simulink library "InfrastructureVariants_CL"  (R2020a)
settings: Solver=VariableStepAuto  StartTime=0.0  StopTime=10.0  RelTol=1e-3
undefined symbols (not defined in the file): Buffer, ENV, Int, Int_ran, route, TRAN, VEH
(part 1 of 2)
settings Model: Creator=John Jr  LastModifiedBy=John Jr
settings DataIOCC: ReturnWorkspaceOutputs=off
settings DebuggingCC: ArithmeticOperatorsInVariantConditions=warning
settings SFSimCC: CustomCodeUndefinedFunction=UseInterfaceOnly

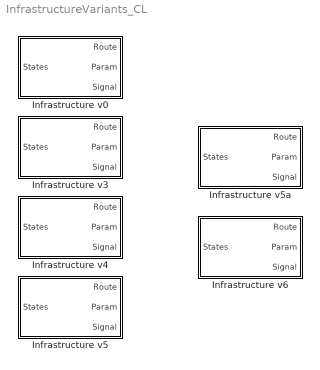
== system InfrastructureVariants_CL ==
  Infrastructure v0 : Subsystem
      mask Display:
      | patch([0 1 1 0], [0 0 1 1],[1 .8 1])
      | 
      | port_label('input',1,'States')
      | 
      | port_label('output',1,'Route')
      | port_label('output',2,'Param')
      | port_label('output',3,'Signal')
  Infrastructure v3 : Subsystem
      mask Display:
      | patch([0 1 1 0], [0 0 1 1],[1 .8 1])
      | 
      | port_label('input',1,'States')
      | 
      | port_label('output',1,'Route')
      | port_label('output',2,'Param')
      | port_label('output',3,'Signal')
  Infrastructure v4 : Subsystem
      mask Display:
      | patch([0 1 1 0], [0 0 1 1],[1 .8 1])
      | 
      | port_label('input',1,'States')
      | 
      | port_label('output',1,'Route')
      | port_label('output',2,'Param')
      | port_label('output',3,'Signal')
  Infrastructure v5 : Subsystem
      mask Display:
      | patch([0 1 1 0], [0 0 1 1],[1 .8 1])
      | 
      | port_label('input',1,'States')
      | 
      | port_label('output',1,'Route')
      | port_label('output',2,'Param')
      | port_label('output',3,'Signal')
  Infrastructure v5a : Subsystem
      mask Display:
      | patch([0 1 1 0], [0 0 1 1],[1 .8 1])
      | 
      | port_label('input',1,'States')
      | 
      | port_label('output',1,'Route')
      | port_label('output',2,'Param')
      | port_label('output',3,'Signal')
  Infrastructure v6 : Subsystem
      mask Display:
      | patch([0 1 1 0], [0 0 1 1],[1 .8 1])
      | 
      | port_label('input',1,'States')
      | 
      | port_label('output',1,'Route')
      | port_label('output',2,'Param')
      | port_label('output',3,'Signal')

== system InfrastructureVariants_CL/Infrastructure v0 ==
  States : Inport
  Route Generator : Subsystem
  Signal Info v5 : Subsystem
      mask Display:
      | patch([0 1 1 0], [0 0 1 1],[.8 1 1])
      | 
      | port_label('input',1,'States')
      | 
      | port_label('output',1,'Signal')
  Veh Param : Subsystem
  Route : Outport  VectorParamsAs1DForOutWhenUnconnected=off
  Param : Outport  Port=2  VectorParamsAs1DForOutWhenUnconnected=off
  Signal : Outport  Port=3  VectorParamsAs1DForOutWhenUnconnected=off
  wires:
  States/1 -> Signal Info v5/1(In1)
  Route Generator/1(Route Info) -> Route/1
  Veh Param/1(Param) -> Param/1
  Signal Info v5/1(Out1) -> Signal/1

== system InfrastructureVariants_CL/Infrastructure v3 ==
  States : Inport
  Route Generator : Subsystem
  Signal Info v3 : Subsystem
      mask Display:
      | patch([0 1 1 0], [0 0 1 1],[.8 1 1])
      | 
      | port_label('input',1,'States')
      | 
      | port_label('output',1,'Signal')
  Veh Param : Subsystem
  Route : Outport  VectorParamsAs1DForOutWhenUnconnected=off
  Param : Outport  Port=2  VectorParamsAs1DForOutWhenUnconnected=off
  Signal : Outport  Port=3  VectorParamsAs1DForOutWhenUnconnected=off
  wires:
  States/1 -> Signal Info v3/1(In1)
  Route Generator/1(Route Info) -> Route/1
  Veh Param/1(Param) -> Param/1
  Signal Info v3/1(Out1) -> Signal/1

== system InfrastructureVariants_CL/Infrastructure v4 ==
  States : Inport
  Route Generator : Subsystem
  Signal Info v4 : Subsystem
      mask Display:
      | patch([0 1 1 0], [0 0 1 1],[.8 1 1])
      | 
      | port_label('input',1,'States')
      | 
      | port_label('output',1,'Signal')
  Veh Param : Subsystem
  Route : Outport  VectorParamsAs1DForOutWhenUnconnected=off
  Param : Outport  Port=2  VectorParamsAs1DForOutWhenUnconnected=off
  Signal : Outport  Port=3  VectorParamsAs1DForOutWhenUnconnected=off
  wires:
  States/1 -> Signal Info v4/1(In1)
  Route Generator/1(Route Info) -> Route/1
  Veh Param/1(Param) -> Param/1
  Signal Info v4/1(Out1) -> Signal/1

== system InfrastructureVariants_CL/Infrastructure v5 ==
  States : Inport
  Route Generator : Subsystem
  Signal Info v5 : Subsystem
      mask Display:
      | patch([0 1 1 0], [0 0 1 1],[.8 1 1])
      | 
      | port_label('input',1,'States')
      | 
      | port_label('output',1,'Signal')
  Veh Param : Subsystem
  Route : Outport  VectorParamsAs1DForOutWhenUnconnected=off
  Param : Outport  Port=2  VectorParamsAs1DForOutWhenUnconnected=off
  Signal : Outport  Port=3  VectorParamsAs1DForOutWhenUnconnected=off
  wires:
  States/1 -> Signal Info v5/1(In1)
  Route Generator/1(Route Info) -> Route/1
  Veh Param/1(Param) -> Param/1
  Signal Info v5/1(Out1) -> Signal/1

== system InfrastructureVariants_CL/Infrastructure v5a ==
  States : Inport
  Route Generator : Subsystem
  Signal Info v5a : Subsystem
      mask Display:
      | patch([0 1 1 0], [0 0 1 1],[.8 1 1])
      | 
      | port_label('input',1,'States')
      | 
      | port_label('output',1,'Signal')
  Veh Param : Subsystem
  Route : Outport  VectorParamsAs1DForOutWhenUnconnected=off
  Param : Outport  Port=2  VectorParamsAs1DForOutWhenUnconnected=off
  Signal : Outport  Port=3  VectorParamsAs1DForOutWhenUnconnected=off
  wires:
  States/1 -> Signal Info v5a/1(In1)
  Route Generator/1(Route Info) -> Route/1
  Veh Param/1(Param) -> Param/1
  Signal Info v5a/1(Out1) -> Signal/1

== system InfrastructureVariants_CL/Infrastructure v6 ==
  States : Inport
  Route Generator : Subsystem
  Signal Info v5 : Subsystem
      mask Display:
      | patch([0 1 1 0], [0 0 1 1],[.8 1 1])
      | 
      | port_label('input',1,'States')
      | 
      | port_label('output',1,'Signal')
  Veh Param : Subsystem
  Route : Outport  VectorParamsAs1DForOutWhenUnconnected=off
  Param : Outport  Port=2  VectorParamsAs1DForOutWhenUnconnected=off
  Signal : Outport  Port=3  VectorParamsAs1DForOutWhenUnconnected=off
  wires:
  States/1 -> Signal Info v5/1(In1)
  Route Generator/1(Route Info) -> Route/1
  Veh Param/1(Param) -> Param/1
  Signal Info v5/1(Out1) -> Signal/1

== system InfrastructureVariants_CL/Infrastructure v0/Route Generator ==
  Constant1 : Constant  Value=route
  Route Info : Outport  VectorParamsAs1DForOutWhenUnconnected=off
  wires:
  Constant1/1 -> Route Info/1  "route"

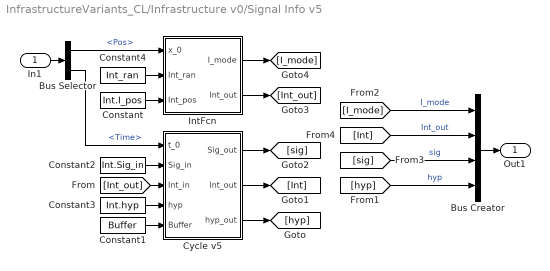
== system InfrastructureVariants_CL/Infrastructure v0/Signal Info v5 ==
  In1 : Inport
  Bus Creator : BusCreator  Inputs=4
  Bus Selector : BusSelector  OutputSignals=Pos,Time
  Constant : Constant  Value=Int.I_pos
  Constant1 : Constant  Value=Buffer
  Constant2 : Constant  Value=Int.Sig_in
  Constant3 : Constant  Value=Int.hyp
  Constant4 : Constant  Value=Int_ran
  Cycle v5 : MATLAB Function  TreatAsAtomicUnit=on
  IntFcn : MATLAB Function  TreatAsAtomicUnit=on
  Out1 : Outport  VectorParamsAs1DForOutWhenUnconnected=off
  wires:
  Constant1/1 -> Cycle v5/5(Buffer)
  Cycle v5/3(hyp_out) -> [hyp]
  Cycle v5/2(Int_out) -> [Int]
  Cycle v5/1(Sig_out) -> [sig]
  [sig] -> Bus Creator/3  "sig"
  [hyp] -> Bus Creator/4  "hyp"
  Bus Creator/1 -> Out1/1
  Constant3/1 -> Cycle v5/4(hyp)
  Constant4/1 -> IntFcn/2(Int_ran)
  [Int_out] -> Cycle v5/3(Int_in)
  IntFcn/2(Int_out) -> [Int_out]
  [Int] -> Bus Creator/2  "Int_out"
  Constant/1 -> IntFcn/3(Int_pos)
  IntFcn/1(I_mode) -> [I_mode]
  [I_mode] -> Bus Creator/1  "I_mode"
  Constant2/1 -> Cycle v5/2(Sig_in)
  In1/1 -> Bus Selector/1
  Bus Selector/1 -> IntFcn/1(x_0)  "<Pos>"
  Bus Selector/2 -> Cycle v5/1(t_0)  "<Time>"

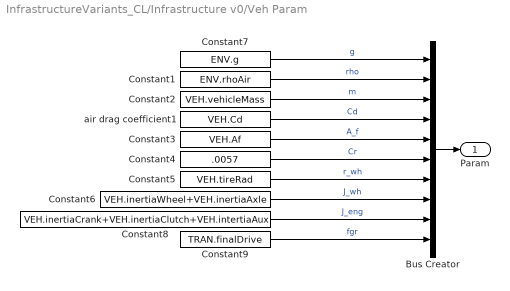
== system InfrastructureVariants_CL/Infrastructure v0/Veh Param ==
  Bus Creator : BusCreator  Inputs=10
  Constant1 : Constant  Value=ENV.rhoAir
  Constant2 : Constant  Value=VEH.vehicleMass
  Constant3 : Constant  Value=VEH.Af
  Constant4 : Constant  Value=.0057
  Constant5 : Constant  Value=VEH.tireRad
  Constant6 : Constant  Value=VEH.inertiaWheel+VEH.inertiaAxle
  Constant7 : Constant  Value=ENV.g
  Constant8 : Constant  Value=VEH.inertiaCrank+VEH.inertiaClutch+VEH.intertiaAux
  Constant9 : Constant  Value=TRAN.finalDrive
  air drag coefficient1 : Constant  Value=VEH.Cd
  Param : Outport  VectorParamsAs1DForOutWhenUnconnected=off
  wires:
  Bus Creator/1 -> Param/1
  Constant7/1 -> Bus Creator/1  "g"
  Constant1/1 -> Bus Creator/2  "rho"
  Constant2/1 -> Bus Creator/3  "m"
  Constant3/1 -> Bus Creator/5  "A_f"
  Constant4/1 -> Bus Creator/6  "Cr"
  Constant5/1 -> Bus Creator/7  "r_wh"
  Constant9/1 -> Bus Creator/10  "fgr"
  air drag coefficient1/1 -> Bus Creator/4  "Cd"
  Constant6/1 -> Bus Creator/8  "J_wh"
  Constant8/1 -> Bus Creator/9  "J_eng"

== system InfrastructureVariants_CL/Infrastructure v3/Route Generator ==
  Constant1 : Constant  Value=route
  Route Info : Outport  VectorParamsAs1DForOutWhenUnconnected=off
  wires:
  Constant1/1 -> Route Info/1  "route"

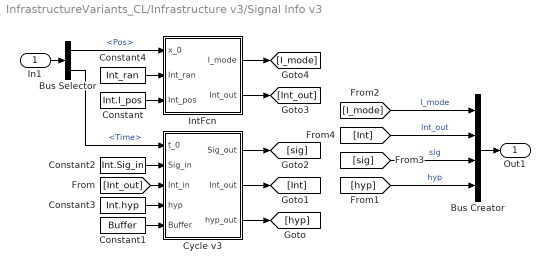
== system InfrastructureVariants_CL/Infrastructure v3/Signal Info v3 ==
  In1 : Inport
  Bus Creator : BusCreator  Inputs=4
  Bus Selector : BusSelector  OutputSignals=Pos,Time
  Constant : Constant  Value=Int.I_pos
  Constant1 : Constant  Value=Buffer
  Constant2 : Constant  Value=Int.Sig_in
  Constant3 : Constant  Value=Int.hyp
  Constant4 : Constant  Value=Int_ran
  Cycle v3 : MATLAB Function  TreatAsAtomicUnit=on
  IntFcn : MATLAB Function  TreatAsAtomicUnit=on
  Out1 : Outport  VectorParamsAs1DForOutWhenUnconnected=off
  wires:
  Constant1/1 -> Cycle v3/5(Buffer)
  Cycle v3/3(hyp_out) -> [hyp]
  Cycle v3/2(Int_out) -> [Int]
  Cycle v3/1(Sig_out) -> [sig]
  [sig] -> Bus Creator/3  "sig"
  [hyp] -> Bus Creator/4  "hyp"
  Bus Creator/1 -> Out1/1
  Constant3/1 -> Cycle v3/4(hyp)
  Constant4/1 -> IntFcn/2(Int_ran)
  [Int_out] -> Cycle v3/3(Int_in)
  IntFcn/2(Int_out) -> [Int_out]
  [Int] -> Bus Creator/2  "Int_out"
  Constant/1 -> IntFcn/3(Int_pos)
  IntFcn/1(I_mode) -> [I_mode]
  [I_mode] -> Bus Creator/1  "I_mode"
  Constant2/1 -> Cycle v3/2(Sig_in)
  In1/1 -> Bus Selector/1
  Bus Selector/1 -> IntFcn/1(x_0)  "<Pos>"
  Bus Selector/2 -> Cycle v3/1(t_0)  "<Time>"

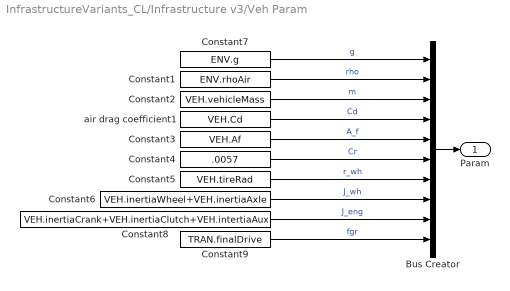
== system InfrastructureVariants_CL/Infrastructure v3/Veh Param ==
  Bus Creator : BusCreator  Inputs=10
  Constant1 : Constant  Value=ENV.rhoAir
  Constant2 : Constant  Value=VEH.vehicleMass
  Constant3 : Constant  Value=VEH.Af
  Constant4 : Constant  Value=.0057
  Constant5 : Constant  Value=VEH.tireRad
  Constant6 : Constant  Value=VEH.inertiaWheel+VEH.inertiaAxle
  Constant7 : Constant  Value=ENV.g
  Constant8 : Constant  Value=VEH.inertiaCrank+VEH.inertiaClutch+VEH.intertiaAux
  Constant9 : Constant  Value=TRAN.finalDrive
  air drag coefficient1 : Constant  Value=VEH.Cd
  Param : Outport  VectorParamsAs1DForOutWhenUnconnected=off
  wires:
  Bus Creator/1 -> Param/1
  Constant7/1 -> Bus Creator/1  "g"
  Constant1/1 -> Bus Creator/2  "rho"
  Constant2/1 -> Bus Creator/3  "m"
  Constant3/1 -> Bus Creator/5  "A_f"
  Constant4/1 -> Bus Creator/6  "Cr"
  Constant5/1 -> Bus Creator/7  "r_wh"
  Constant9/1 -> Bus Creator/10  "fgr"
  air drag coefficient1/1 -> Bus Creator/4  "Cd"
  Constant6/1 -> Bus Creator/8  "J_wh"
  Constant8/1 -> Bus Creator/9  "J_eng"

== system InfrastructureVariants_CL/Infrastructure v4/Route Generator ==
  Constant1 : Constant  Value=route
  Route Info : Outport  VectorParamsAs1DForOutWhenUnconnected=off
  wires:
  Constant1/1 -> Route Info/1  "route"

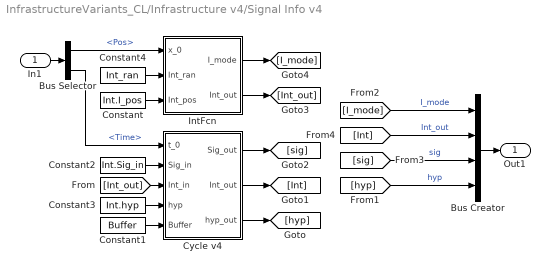
== system InfrastructureVariants_CL/Infrastructure v4/Signal Info v4 ==
  In1 : Inport
  Bus Creator : BusCreator  Inputs=4
  Bus Selector : BusSelector  OutputSignals=Pos,Time
  Constant : Constant  Value=Int.I_pos
  Constant1 : Constant  Value=Buffer
  Constant2 : Constant  Value=Int.Sig_in
  Constant3 : Constant  Value=Int.hyp
  Constant4 : Constant  Value=Int_ran
  Cycle v4 : MATLAB Function  TreatAsAtomicUnit=on
  IntFcn : MATLAB Function  TreatAsAtomicUnit=on
  Out1 : Outport  VectorParamsAs1DForOutWhenUnconnected=off
  wires:
  Constant1/1 -> Cycle v4/5(Buffer)
  Cycle v4/3(hyp_out) -> [hyp]
  Cycle v4/2(Int_out) -> [Int]
  Cycle v4/1(Sig_out) -> [sig]
  [sig] -> Bus Creator/3  "sig"
  [hyp] -> Bus Creator/4  "hyp"
  Bus Creator/1 -> Out1/1
  Constant3/1 -> Cycle v4/4(hyp)
  Constant4/1 -> IntFcn/2(Int_ran)
  [Int_out] -> Cycle v4/3(Int_in)
  IntFcn/2(Int_out) -> [Int_out]
  [Int] -> Bus Creator/2  "Int_out"
  Constant/1 -> IntFcn/3(Int_pos)
  IntFcn/1(I_mode) -> [I_mode]
  [I_mode] -> Bus Creator/1  "I_mode"
  Constant2/1 -> Cycle v4/2(Sig_in)
  In1/1 -> Bus Selector/1
  Bus Selector/1 -> IntFcn/1(x_0)  "<Pos>"
  Bus Selector/2 -> Cycle v4/1(t_0)  "<Time>"

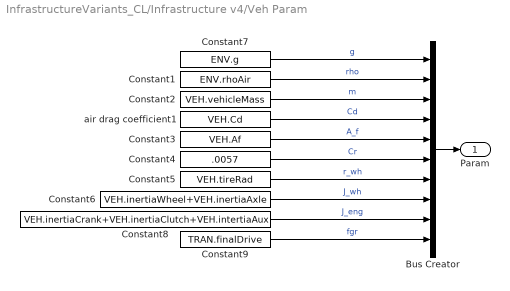
== system InfrastructureVariants_CL/Infrastructure v4/Veh Param ==
  Bus Creator : BusCreator  Inputs=10
  Constant1 : Constant  Value=ENV.rhoAir
  Constant2 : Constant  Value=VEH.vehicleMass
  Constant3 : Constant  Value=VEH.Af
  Constant4 : Constant  Value=.0057
  Constant5 : Constant  Value=VEH.tireRad
  Constant6 : Constant  Value=VEH.inertiaWheel+VEH.inertiaAxle
  Constant7 : Constant  Value=ENV.g
  Constant8 : Constant  Value=VEH.inertiaCrank+VEH.inertiaClutch+VEH.intertiaAux
  Constant9 : Constant  Value=TRAN.finalDrive
  air drag coefficient1 : Constant  Value=VEH.Cd
  Param : Outport  VectorParamsAs1DForOutWhenUnconnected=off
  wires:
  Bus Creator/1 -> Param/1
  Constant7/1 -> Bus Creator/1  "g"
  Constant1/1 -> Bus Creator/2  "rho"
  Constant2/1 -> Bus Creator/3  "m"
  Constant3/1 -> Bus Creator/5  "A_f"
  Constant4/1 -> Bus Creator/6  "Cr"
  Constant5/1 -> Bus Creator/7  "r_wh"
  Constant9/1 -> Bus Creator/10  "fgr"
  air drag coefficient1/1 -> Bus Creator/4  "Cd"
  Constant6/1 -> Bus Creator/8  "J_wh"
  Constant8/1 -> Bus Creator/9  "J_eng"

== system InfrastructureVariants_CL/Infrastructure v5/Route Generator ==
  Constant1 : Constant  Value=route
  Route Info : Outport  VectorParamsAs1DForOutWhenUnconnected=off
  wires:
  Constant1/1 -> Route Info/1  "route"

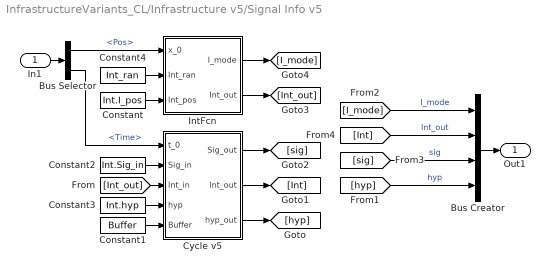
== system InfrastructureVariants_CL/Infrastructure v5/Signal Info v5 ==
  In1 : Inport
  Bus Creator : BusCreator  Inputs=4
  Bus Selector : BusSelector  OutputSignals=Pos,Time
  Constant : Constant  Value=Int.I_pos
  Constant1 : Constant  Value=Buffer
  Constant2 : Constant  Value=Int.Sig_in
  Constant3 : Constant  Value=Int.hyp
  Constant4 : Constant  Value=Int_ran
  Cycle v5 : MATLAB Function  TreatAsAtomicUnit=on
  IntFcn : MATLAB Function  TreatAsAtomicUnit=on
  Out1 : Outport  VectorParamsAs1DForOutWhenUnconnected=off
  wires:
  Constant1/1 -> Cycle v5/5(Buffer)
  Cycle v5/3(hyp_out) -> [hyp]
  Cycle v5/2(Int_out) -> [Int]
  Cycle v5/1(Sig_out) -> [sig]
  [sig] -> Bus Creator/3  "sig"
  [hyp] -> Bus Creator/4  "hyp"
  Bus Creator/1 -> Out1/1
  Constant3/1 -> Cycle v5/4(hyp)
  Constant4/1 -> IntFcn/2(Int_ran)
  [Int_out] -> Cycle v5/3(Int_in)
  IntFcn/2(Int_out) -> [Int_out]
  [Int] -> Bus Creator/2  "Int_out"
  Constant/1 -> IntFcn/3(Int_pos)
  IntFcn/1(I_mode) -> [I_mode]
  [I_mode] -> Bus Creator/1  "I_mode"
  Constant2/1 -> Cycle v5/2(Sig_in)
  In1/1 -> Bus Selector/1
  Bus Selector/1 -> IntFcn/1(x_0)  "<Pos>"
  Bus Selector/2 -> Cycle v5/1(t_0)  "<Time>"

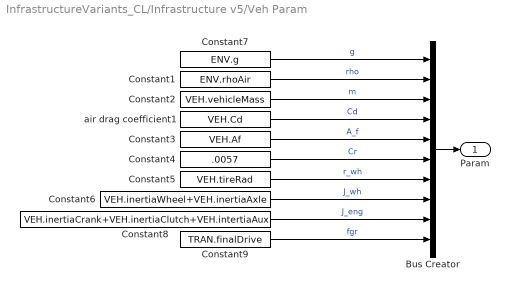
== system InfrastructureVariants_CL/Infrastructure v5/Veh Param ==
  Bus Creator : BusCreator  Inputs=10
  Constant1 : Constant  Value=ENV.rhoAir
  Constant2 : Constant  Value=VEH.vehicleMass
  Constant3 : Constant  Value=VEH.Af
  Constant4 : Constant  Value=.0057
  Constant5 : Constant  Value=VEH.tireRad
  Constant6 : Constant  Value=VEH.inertiaWheel+VEH.inertiaAxle
  Constant7 : Constant  Value=ENV.g
  Constant8 : Constant  Value=VEH.inertiaCrank+VEH.inertiaClutch+VEH.intertiaAux
  Constant9 : Constant  Value=TRAN.finalDrive
  air drag coefficient1 : Constant  Value=VEH.Cd
  Param : Outport  VectorParamsAs1DForOutWhenUnconnected=off
  wires:
  Bus Creator/1 -> Param/1
  Constant7/1 -> Bus Creator/1  "g"
  Constant1/1 -> Bus Creator/2  "rho"
  Constant2/1 -> Bus Creator/3  "m"
  Constant3/1 -> Bus Creator/5  "A_f"
  Constant4/1 -> Bus Creator/6  "Cr"
  Constant5/1 -> Bus Creator/7  "r_wh"
  Constant9/1 -> Bus Creator/10  "fgr"
  air drag coefficient1/1 -> Bus Creator/4  "Cd"
  Constant6/1 -> Bus Creator/8  "J_wh"
  Constant8/1 -> Bus Creator/9  "J_eng"

== system InfrastructureVariants_CL/Infrastructure v5a/Route Generator ==
  Constant1 : Constant  Value=route
  Route Info : Outport  VectorParamsAs1DForOutWhenUnconnected=off
  wires:
  Constant1/1 -> Route Info/1  "route"

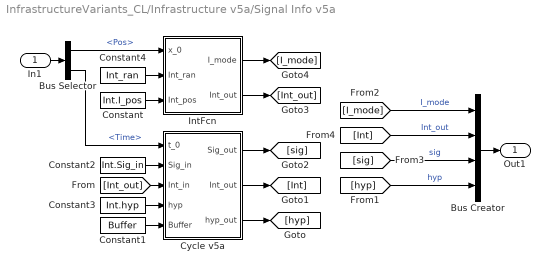
== system InfrastructureVariants_CL/Infrastructure v5a/Signal Info v5a ==
  In1 : Inport
  Bus Creator : BusCreator  Inputs=4
  Bus Selector : BusSelector  OutputSignals=Pos,Time
  Constant : Constant  Value=Int.I_pos
  Constant1 : Constant  Value=Buffer
  Constant2 : Constant  Value=Int.Sig_in
  Constant3 : Constant  Value=Int.hyp
  Constant4 : Constant  Value=Int_ran
  Cycle v5a : MATLAB Function  TreatAsAtomicUnit=on
  IntFcn : MATLAB Function  TreatAsAtomicUnit=on
  Out1 : Outport  VectorParamsAs1DForOutWhenUnconnected=off
  wires:
  Constant1/1 -> Cycle v5a/5(Buffer)
  Cycle v5a/3(hyp_out) -> [hyp]
  Cycle v5a/2(Int_out) -> [Int]
  Cycle v5a/1(Sig_out) -> [sig]
  [sig] -> Bus Creator/3  "sig"
  [hyp] -> Bus Creator/4  "hyp"
  Bus Creator/1 -> Out1/1
  Constant3/1 -> Cycle v5a/4(hyp)
  Constant4/1 -> IntFcn/2(Int_ran)
  [Int_out] -> Cycle v5a/3(Int_in)
  IntFcn/2(Int_out) -> [Int_out]
  [Int] -> Bus Creator/2  "Int_out"
  Constant/1 -> IntFcn/3(Int_pos)
  IntFcn/1(I_mode) -> [I_mode]
  [I_mode] -> Bus Creator/1  "I_mode"
  Constant2/1 -> Cycle v5a/2(Sig_in)
  In1/1 -> Bus Selector/1
  Bus Selector/1 -> IntFcn/1(x_0)  "<Pos>"
  Bus Selector/2 -> Cycle v5a/1(t_0)  "<Time>"

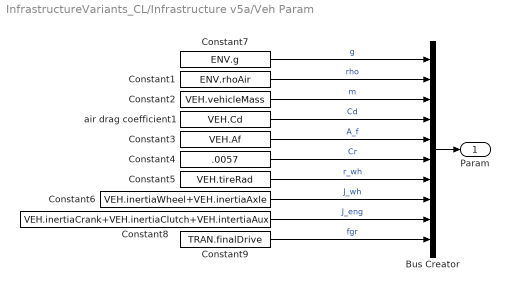
== system InfrastructureVariants_CL/Infrastructure v5a/Veh Param ==
  Bus Creator : BusCreator  Inputs=10
  Constant1 : Constant  Value=ENV.rhoAir
  Constant2 : Constant  Value=VEH.vehicleMass
  Constant3 : Constant  Value=VEH.Af
  Constant4 : Constant  Value=.0057
  Constant5 : Constant  Value=VEH.tireRad
  Constant6 : Constant  Value=VEH.inertiaWheel+VEH.inertiaAxle
  Constant7 : Constant  Value=ENV.g
  Constant8 : Constant  Value=VEH.inertiaCrank+VEH.inertiaClutch+VEH.intertiaAux
  Constant9 : Constant  Value=TRAN.finalDrive
  air drag coefficient1 : Constant  Value=VEH.Cd
  Param : Outport  VectorParamsAs1DForOutWhenUnconnected=off
  wires:
  Bus Creator/1 -> Param/1
  Constant7/1 -> Bus Creator/1  "g"
  Constant1/1 -> Bus Creator/2  "rho"
  Constant2/1 -> Bus Creator/3  "m"
  Constant3/1 -> Bus Creator/5  "A_f"
  Constant4/1 -> Bus Creator/6  "Cr"
  Constant5/1 -> Bus Creator/7  "r_wh"
  Constant9/1 -> Bus Creator/10  "fgr"
  air drag coefficient1/1 -> Bus Creator/4  "Cd"
  Constant6/1 -> Bus Creator/8  "J_wh"
  Constant8/1 -> Bus Creator/9  "J_eng"

== system InfrastructureVariants_CL/Infrastructure v6/Route Generator ==
  Constant1 : Constant  Value=route
  Route Info : Outport  VectorParamsAs1DForOutWhenUnconnected=off
  wires:
  Constant1/1 -> Route Info/1  "route"

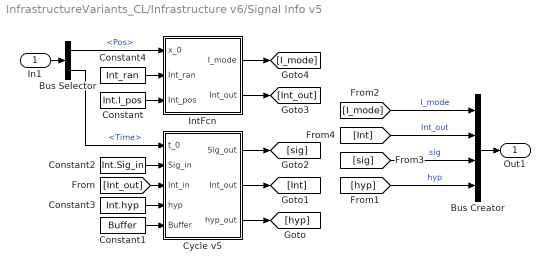
== system InfrastructureVariants_CL/Infrastructure v6/Signal Info v5 ==
  In1 : Inport
  Bus Creator : BusCreator  Inputs=4
  Bus Selector : BusSelector  OutputSignals=Pos,Time
  Constant : Constant  Value=Int.I_pos
  Constant1 : Constant  Value=Buffer
  Constant2 : Constant  Value=Int.Sig_in
  Constant3 : Constant  Value=Int.hyp
  Constant4 : Constant  Value=Int_ran
  Cycle v5 : MATLAB Function  TreatAsAtomicUnit=on
  IntFcn : MATLAB Function  TreatAsAtomicUnit=on
  Out1 : Outport  VectorParamsAs1DForOutWhenUnconnected=off
  wires:
  Constant1/1 -> Cycle v5/5(Buffer)
  Cycle v5/3(hyp_out) -> [hyp]
  Cycle v5/2(Int_out) -> [Int]
  Cycle v5/1(Sig_out) -> [sig]
  [sig] -> Bus Creator/3  "sig"
  [hyp] -> Bus Creator/4  "hyp"
  Bus Creator/1 -> Out1/1
  Constant3/1 -> Cycle v5/4(hyp)
  Constant4/1 -> IntFcn/2(Int_ran)
  [Int_out] -> Cycle v5/3(Int_in)
  IntFcn/2(Int_out) -> [Int_out]
  [Int] -> Bus Creator/2  "Int_out"
  Constant/1 -> IntFcn/3(Int_pos)
  IntFcn/1(I_mode) -> [I_mode]
  [I_mode] -> Bus Creator/1  "I_mode"
  Constant2/1 -> Cycle v5/2(Sig_in)
  In1/1 -> Bus Selector/1
  Bus Selector/1 -> IntFcn/1(x_0)  "<Pos>"
  Bus Selector/2 -> Cycle v5/1(t_0)  "<Time>"

== system InfrastructureVariants_CL/Infrastructure v6/Veh Param ==
  Bus Creator : BusCreator  Inputs=10
  Constant1 : Constant  Value=ENV.rhoAir
  Constant2 : Constant  Value=VEH.vehicleMass
  Constant3 : Constant  Value=VEH.Af
  Constant4 : Constant  Value=.0057
  Constant5 : Constant  Value=VEH.tireRad
  Constant6 : Constant  Value=VEH.inertiaWheel+VEH.inertiaAxle
  Constant7 : Constant  Value=ENV.g
  Constant8 : Constant  Value=VEH.inertiaCrank+VEH.inertiaClutch+VEH.intertiaAux
  Constant9 : Constant  Value=TRAN.finalDrive
  air drag coefficient1 : Constant  Value=VEH.Cd
  Param : Outport  VectorParamsAs1DForOutWhenUnconnected=off
  wires:
  Bus Creator/1 -> Param/1
  Constant7/1 -> Bus Creator/1  "g"
  Constant1/1 -> Bus Creator/2  "rho"
  Constant2/1 -> Bus Creator/3  "m"
  Constant3/1 -> Bus Creator/5  "A_f"
  Constant4/1 -> Bus Creator/6  "Cr"
  Constant5/1 -> Bus Creator/7  "r_wh"
  Constant9/1 -> Bus Creator/10  "fgr"
  air drag coefficient1/1 -> Bus Creator/4  "Cd"
  Constant6/1 -> Bus Creator/8  "J_wh"
  Constant8/1 -> Bus Creator/9  "J_eng"

== matlab function InfrastructureVariants_CL/Infrastructure v6/Signal Info v5/Cycle v5 ==
  data: Sig_out output; Int_out output; t_0 input; Sig_in input; Int_in input; hyp_out output; hyp input; Buffer input
function [Sig_out,Int_out,hyp_out] = fcn(t_0,Sig_in,Int_in,hyp,Buffer)

Int_cur = Int_in(~isnan(Int_in(:,1)),1);        %   Current intersections within communication range
Cs = Sig_in(:,:,1);                             %   s - Signal cycle start times
G = Sig_in(:,:,3);                              %   s - Signal green phase length 
R = Sig_in(:,:,4);                              %   s - Signal red phase length 
Y = Buffer(:,1);                                %   s - Signal yellow length
Rc = Buffer(:,2);                               %   s - Signal red clearance length 
N = 10;                                         %   # of upcoming intersections 
M = 20;                                         %   Size of intersection data queue
idx = zeros(N,1);                               %   Initialize current cycle index vector
Sig_out = NaN*ones(N,M,4);                      %   Initialize cycle length output 
hyp_out = NaN*ones(N,3,2);                      %   Initialize hyperparameter output 
T_0 = NaN*ones(N,1);                            %   Initialize current cycle start time output
L_0 = NaN*ones(N,1);                            %   Initialize light status flag
B_0 = NaN*ones(N,1);                            %   Initialize yellow light length 
for i = 1:length(Int_cur)
    idx(i) = find(Cs(Int_cur(i),:) <= t_0,1,'last');        %   Find current cycle for upcoming intersections 
    tR = Cs(Int_cur(i),idx(i))+G(Int_cur(i),idx(i));        %   s - Time at which light turns red
    tL1 = tR-t_0;                                           %   s - Time left until red
    tL2 = Cs(Int_cur(i),idx(i)+1)-t_0;                      %   s - Time left until green
    if tL1 > Y(Int_cur(i))*2 
        L_0(i) = 0;                                         %   Light is green and time left is unknown 
        Sig_out(i,:,3) = idx(i)-M:idx(i)-1;                 %   Available green phase lengths
        Sig_out(i,:,4) = idx(i)-M:idx(i)-1;                 %   Available red phase lengths
    elseif tL1 <= Y(Int_cur(i))*2 && tL1 > 0
        L_0(i) = 1;                                         %   Light is green and time left is known 
        Sig_out(i,:,3) = idx(i)-M+1:idx(i);                 %   Available green phase lengths
        Sig_out(i,:,4) = idx(i)-M:idx(i)-1;                 %   Available red phase lengths
    elseif tL2 > (Y(Int_cur(i))+Rc(Int_cur(i)))*2 
        L_0(i) = 2;                                         %   Light is red and time left is unknown 
        Sig_out(i,:,3) = idx(i)-M+1:idx(i);                 %   Available green phase lengths
        Sig_out(i,:,4) = idx(i)-M:idx(i)-1;                 %   Available red phase lengths
    else           
        L_0(i) = 3;                                         %   Light is red and time left is known 
        Sig_out(i,:,3) = idx(i)-M+1:idx(i);                 %   Available green phase lengths
        Sig_out(i,:,4) = idx(i)-M+1:idx(i);                 %   Available red phase lengths
    end
    B_0(i) = 2*Y(Int_cur(i));                               %   Yellow light length for upcoming intersections 
    Sig_out(i,:,1) = G(Int_cur(i),Sig_out(i,:,3));          %   Create a vector with the past green phase lengths
    Sig_out(i,:,2) = R(Int_cur(i),Sig_out(i,:,4));          %   Create a vector with the past red phase lengths
    T_0(i) = Cs(Int_cur(i),idx(i));                         %   Current cycle start time
    hypG1 = var(Sig_out(i,:,1));
    hypR1 = var(Sig_out(i,:,2));
    hyp_out(i,:,1) = [hypG1 1 .0625];                       %   Get relevant hyperparameters 
    hyp_out(i,:,2) = [hypR1 1 .0625];                       %   Get relevant hyperparameters 
end
Int_out = [Int_in, T_0, L_0, B_0];                          %   Update intersection variables

== matlab function InfrastructureVariants_CL/Infrastructure v6/Signal Info v5/IntFcn ==
  data: x_0 input; I_mode output; Int_ran input; Int_pos input; Int_out output
function [I_mode,Int_out]  = fcn(x_0,Int_ran,Int_pos)

Int_pos = Int_pos(:,1);                         %   Intersection Positions
[Int_0,~] = find(x_0-Int_pos < 0,1,'first');    %   First intersection within range
[Int_f,~] = find(x_0+Int_ran-Int_pos...         %   Last intersection within range
    > 0,1,'last');
Int_cur = NaN*ones(10,1);                       %   Initialize upcoming intersection vector 
Int_dx = NaN*ones(10,1);                        %   m - Initialize distance to upcoming intersections vector 
Int_gap = NaN*ones(10,1);                       %   m - Initialize distance between intersections vector 
if isempty(Int_0)
    I_mode = 0;                                 %   No upcoming intersection
elseif Int_pos(Int_0(1))-x_0 > Int_ran
    I_mode = 0;                                 %   No upcoming intersection
else
    I_0 = Int_0(1);     I_f = Int_f(1);
    Int_cur(1:I_f-I_0+1,1) = (I_0:I_f)';            %   Upcoming intersections
    I_mode = 1;                                 %   Approaching intersection
    Int_dx(1:I_f-I_0+1,1) = ...                 %   m - Distance to upcoming intersection 
        Int_pos(Int_cur(1:I_f-I_0+1,1))-x_0;
end
Int_gap(1) = Int_dx(1);                         %   m - Distance to first upcoming intersection 
for i = 2:length(Int_gap)
    Int_gap(i) = Int_dx(i)-Int_dx(i-1);         %   m - Distance between further intersections 
end
Int_out = [Int_cur,Int_dx,Int_gap];

== matlab function InfrastructureVariants_CL/Infrastructure v5a/Signal Info v5a/Cycle v5a ==
  data: Sig_out output; Int_out output; t_0 input; Sig_in input; Int_in input; hyp_out output; hyp input; Buffer input
function [Sig_out,Int_out,hyp_out] = fcn(t_0,Sig_in,Int_in,hyp,Buffer)

Int_cur = Int_in(~isnan(Int_in(:,1)),1);        %   Current intersections within communication range
Cs = Sig_in(:,:,1);                             %   s - Signal cycle start times
G = Sig_in(:,:,3);                              %   s - Signal green phase length 
R = Sig_in(:,:,4);                              %   s - Signal red phase length 
Y = Buffer(:,1);                                %   s - Signal yellow length
Rc = Buffer(:,2);                               %   s - Signal red clearance length 
N = 10;                                         %   # of upcoming intersections 
M = 7;                                         %   Size of intersection data queue
idx = zeros(N,1);                               %   Initialize current cycle index vector
Sig_out = NaN*ones(N,M,4);                      %   Initialize cycle length output 
hyp_out = NaN*ones(N,3,2);                      %   Initialize hyperparameter output 
T_0 = NaN*ones(N,1);                            %   Initialize current cycle start time output
L_0 = NaN*ones(N,1);                            %   Initialize light status flag
B_0 = NaN*ones(N,1);                            %   Initialize yellow light length 
for i = 1:length(Int_cur)
    idx(i) = find(Cs(Int_cur(i),:) <= t_0,1,'last');        %   Find current cycle for upcoming intersections 
    B_0(i) = 2*Y(Int_cur(i));                               %   Yellow light length for upcoming intersections 
    Sig_out(i,:,3) = idx(i):idx(i)+M-1;                     %   Available green phase lengths
    Sig_out(i,:,4) = idx(i):idx(i)+M-1;                     %   Available red phase lengths
    Sig_out(i,:,1) = G(Int_cur(i),Sig_out(i,:,3));          %   Create a vector with the past green phase lengths
    Sig_out(i,:,2) = R(Int_cur(i),Sig_out(i,:,4));          %   Create a vector with the past red phase lengths
    T_0(i) = Cs(Int_cur(i),idx(i));                         %   Current cycle start time
    hypG1 = var(Sig_out(i,:,1));
    hypR1 = var(Sig_out(i,:,2));
    hyp_out(i,:,1) = [hypG1 1 .0625];                       %   Get relevant hyperparameters 
    hyp_out(i,:,2) = [hypR1 1 .0625];                       %   Get relevant hyperparameters 
end
Int_out = [Int_in, T_0, L_0, B_0];                          %   Update intersection variables

== matlab function InfrastructureVariants_CL/Infrastructure v5a/Signal Info v5a/IntFcn ==
  data: x_0 input; I_mode output; Int_ran input; Int_pos input; Int_out output
function [I_mode,Int_out]  = fcn(x_0,Int_ran,Int_pos)

Int_pos = Int_pos(:,1);                         %   Intersection Positions
[Int_0,~] = find(x_0-Int_pos < 0,1,'first');    %   First intersection within range
[Int_f,~] = find(x_0+Int_ran-Int_pos...         %   Last intersection within range
    > 0,1,'last');
Int_cur = NaN*ones(10,1);                       %   Initialize upcoming intersection vector 
Int_dx = NaN*ones(10,1);                        %   m - Initialize distance to upcoming intersections vector 
Int_gap = NaN*ones(10,1);                       %   m - Initialize distance between intersections vector 
if isempty(Int_0)
    I_mode = 0;                                 %   No upcoming intersection
elseif Int_pos(Int_0(1))-x_0 > Int_ran
    I_mode = 0;                                 %   No upcoming intersection
else
    I_0 = Int_0(1);     I_f = Int_f(1);
    Int_cur(1:I_f-I_0+1,1) = (I_0:I_f)';            %   Upcoming intersections
    I_mode = 1;                                 %   Approaching intersection
    Int_dx(1:I_f-I_0+1,1) = ...                 %   m - Distance to upcoming intersection 
        Int_pos(Int_cur(1:I_f-I_0+1,1))-x_0;
end
Int_gap(1) = Int_dx(1);                         %   m - Distance to first upcoming intersection 
for i = 2:length(Int_gap)
    Int_gap(i) = Int_dx(i)-Int_dx(i-1);         %   m - Distance between further intersections 
end
Int_out = [Int_cur,Int_dx,Int_gap];

== matlab function InfrastructureVariants_CL/Infrastructure v3/Signal Info v3/IntFcn ==
  data: x_0 input; I_mode output; Int_ran input; Int_pos input; Int_out output
function [I_mode,Int_out]  = fcn(x_0,Int_ran,Int_pos)

Int_pos = Int_pos(:,1);                         %   Intersection Positions
[Int_0,~] = find(x_0-Int_pos < 0,1,'first');    %   First intersection within range
[Int_f,~] = find(x_0+Int_ran-Int_pos...         %   Last intersection within range
    > 0,1,'last');
Int_cur = NaN*ones(10,1);                       %   Initialize upcoming intersection vector 
Int_dx = NaN*ones(10,1);                        %   m - Initialize distance to upcoming intersections vector 
Int_gap = NaN*ones(10,1);                       %   m - Initialize distance between intersections vector 
if isempty(Int_0)
    I_mode = 0;                                 %   No upcoming intersection
elseif Int_pos(Int_0(1))-x_0 > Int_ran
    I_mode = 0;                                 %   No upcoming intersection
else
    I_0 = Int_0(1);     I_f = Int_f(1);
    Int_cur(1:I_f-I_0+1,1) = (I_0:I_f)';            %   Upcoming intersections
    I_mode = 1;                                 %   Approaching intersection
    Int_dx(1:I_f-I_0+1,1) = ...                 %   m - Distance to upcoming intersection 
        Int_pos(Int_cur(1:I_f-I_0+1,1))-x_0;
end
Int_gap(1) = Int_dx(1);                         %   m - Distance to first upcoming intersection 
for i = 2:length(Int_gap)
    Int_gap(i) = Int_dx(i)-Int_dx(i-1);         %   m - Distance between further intersections 
end
Int_out = [Int_cur,Int_dx,Int_gap];

== matlab function InfrastructureVariants_CL/Infrastructure v3/Signal Info v3/Cycle v3 ==
  data: Sig_out output; Int_out output; t_0 input; Sig_in input; Int_in input; hyp_out output; hyp input; Buffer input
function [Sig_out,Int_out,hyp_out] = fcn(t_0,Sig_in,Int_in,hyp,Buffer)

Int_cur = Int_in(~isnan(Int_in(:,1)),1);        %   Find current intersections within range
Cs = Sig_in(:,:,1);                             %   s - Signal cycle start times
G = Sig_in(:,:,3);                              %   s - Signal green phase length 
R = Sig_in(:,:,4);                              %   s - Signal red phase length 
Y = Buffer(:,1);                                %   s - Signal yellow length
Rc = Buffer(:,2);                               %   s - Signal red clearance length 
N = 10;                                         %   # of upcoming intersections 
M = 20;                                         %   Size of intersection data queue
idx = zeros(N,1);                               %   Initialize current cycle index vector
Sig_out = NaN*ones(N,M,2);                      %   Initialize cycle length output 
hyp_out = NaN*ones(N,3,3);                      %   Initialize hyperparameter output 
T_0 = NaN*ones(N,1);                            %   Initialize current cycle start time output
L_0 = NaN*ones(N,1);                            %   Initialize light status flag
for i = 1:length(Int_cur)
    idx(i) = find(Cs(Int_cur(i),:) <= t_0,1,'last');        %   Find current cycle for upcoming intersections 
    tR = Cs(Int_cur(i),idx(i))+G(Int_cur(i),idx(i));        %   s - Time at which light turns red
    tL1 = tR-t_0;                                           %   s - Time left until red
    tL2 = Cs(Int_cur(i),idx(i)+1)-t_0;                      %   s - Time left until green
    if tL1 > Y(Int_cur(i))*2                                %   Light is green and time left is unknown 
        L_0(i) = 0;
    elseif tL1 <= Y(Int_cur(i))*2 && tL1 > 0                %   Light is green and time left is known 
        L_0(i) = 1;
    elseif tL2 > (Y(Int_cur(i))+Rc(Int_cur(i)))*2           %   Light is red and time left is unknown 
        L_0(i) = 2;
    else                                                    %   Light is red and time left is known 
        L_0(i) = 3;
    end
    if L_0(i) == 0
        Sig_out(i,:,1) = G(Int_cur(i),idx(i)-M:idx(i)-1);   %   Create a vector with the past M green phases
    else
        Sig_out(i,:,1) = G(Int_cur(i),idx(i)-M+1:idx(i));   %   Create a vector with the past M-1 green phases and current phase
    end
    if L_0(i) == 3
        Sig_out(i,:,2) = R(Int_cur(i),idx(i)-M+1:idx(i));   %   Create a vector with the past M-1 green phases and current phase
    else
        Sig_out(i,:,2) = R(Int_cur(i),idx(i)-M:idx(i)-1);   %   Create a vector with the past M red phases
    end
    T_0(i) = Cs(Int_cur(i),idx(i));                         %   Current cycle start time
    hyp_out(i,:,:) = hyp(Int_cur(i),:,:,idx(i));            %   Get relevant hyperparameters 
end
Int_out = [Int_in, T_0, L_0];                               %   Update intersection variables

== matlab function InfrastructureVariants_CL/Infrastructure v4/Signal Info v4/Cycle v4 ==
  data: Sig_out output; Int_out output; t_0 input; Sig_in input; Int_in input; hyp_out output; hyp input; Buffer input
function [Sig_out,Int_out,hyp_out] = fcn(t_0,Sig_in,Int_in,hyp,Buffer)

Int_cur = Int_in(isnan(Int_in(:,1))==0,1);      %   Find current intersections within range
Cs = Sig_in(:,:,1);                             %   s - Signal cycle start times
G = Sig_in(:,:,3);                              %   s - Signal green phase length 
Y = Buffer(:,1);                                %   s - Signal yellow length
Rc = Buffer(:,2);                               %   s - Signal red clearance length 
N = 10;                                         %   # of upcoming intersections 
M = 20;                                         %   Size of intersection data queue
idx = zeros(N,1);                               %   Initialize current cycle index vector
Sig_out = NaN*ones(N,M,4);                      %   Initialize cycle length output 
hyp_out = NaN*ones(N,3,2);                      %   Initialize hyperparameter output 
T_0 = NaN*ones(N,1);                            %   Initialize current cycle start time output
L_0 = NaN*ones(N,1);                            %   Initialize light status flag
for i = 1:length(Int_cur)
    idx(i) = find(Cs(Int_cur(i),:) <= t_0,1,'last');        %   Find current cycle for upcoming intersections 
    tR = Cs(Int_cur(i),idx(i))+G(Int_cur(i),idx(i));        %   s - Time at which light turns red
    tL1 = tR-t_0;                                           %   s - Time left until red
    tL2 = Cs(Int_cur(i),idx(i)+1)-t_0;                      %   s - Time left until green
    if tL1 > Y(Int_cur(i))*2 
        L_0(i) = 0;                                         %   Light is green and time left is unknown 
        Sig_out(i,:,3) = idx(i)-M+1:idx(i);                 %   Available green phase start times 
        Sig_out(i,:,4) = idx(i)-M:idx(i)-1;                 %   Available red phase start times 
    elseif tL1 <= Y(Int_cur(i))*2 && tL1 > 0
        L_0(i) = 1;                                         %   Light is green and time left is known 
        Sig_out(i,:,3) = idx(i)-M+1:idx(i);                 %   Available green phase start times 
        Sig_out(i,:,4) = idx(i)-M+1:idx(i);                 %   Available red phase start times 
    elseif tL2 > (Y(Int_cur(i))+Rc(Int_cur(i)))*2 
        L_0(i) = 2;                                         %   Light is red and time left is unknown 
        Sig_out(i,:,3) = idx(i)-M+1:idx(i);                 %   Available green phase start times 
        Sig_out(i,:,4) = idx(i)-M+1:idx(i);                 %   Available red phase start times 
    else           
        L_0(i) = 3;                                         %   Light is red and time left is known 
        Sig_out(i,:,3) = idx(i)-M+2:idx(i)+1;               %   Available green phase start times 
        Sig_out(i,:,4) = idx(i)-M+1:idx(i);                 %   Available red phase start times 
    end
    Sig_out(i,:,1) = Cs(Int_cur(i),Sig_out(i,:,3));         %   Create a vector with the past green phase start times 
    Sig_out(i,:,2) = Cs(Int_cur(i),Sig_out(i,:,4))...       %   Create a vector with the past red phase start times 
        +G(Int_cur(i),Sig_out(i,:,4));      
    T_0(i) = Cs(Int_cur(i),idx(i));                         %   Current cycle start time
    hyp_out(i,:,:) = hyp(Int_cur(i),:,:,idx(i));            %   Get relevant hyperparameters 
end
Int_out = [Int_in, T_0, L_0];                               %   Update intersection variables

== matlab function InfrastructureVariants_CL/Infrastructure v4/Signal Info v4/IntFcn ==
  data: x_0 input; I_mode output; Int_ran input; Int_pos input; Int_out output
function [I_mode,Int_out]  = fcn(x_0,Int_ran,Int_pos)

Int_pos = Int_pos(:,1);                         %   Intersection Positions
[Int_0,~] = find(x_0-Int_pos < 0,1,'first');    %   First intersection within range
[Int_f,~] = find(x_0+Int_ran-Int_pos...         %   Last intersection within range
    > 0,1,'last');
Int_cur = NaN*ones(10,1);                       %   Initialize upcoming intersection vector 
Int_dx = NaN*ones(10,1);                        %   m - Initialize distance to upcoming intersections vector 
Int_gap = NaN*ones(10,1);                       %   m - Initialize distance between intersections vector 
if isempty(Int_0)
    I_mode = 0;                                 %   No upcoming intersection
elseif Int_pos(Int_0(1))-x_0 > Int_ran
    I_mode = 0;                                 %   No upcoming intersection
else
    I_0 = Int_0(1);     I_f = Int_f(1);
    Int_cur(1:I_f-I_0+1,1) = (I_0:I_f)';            %   Upcoming intersections
    I_mode = 1;                                 %   Approaching intersection
    Int_dx(1:I_f-I_0+1,1) = ...                 %   m - Distance to upcoming intersection 
        Int_pos(Int_cur(1:I_f-I_0+1,1))-x_0;
end
Int_gap(1) = Int_dx(1);                         %   m - Distance to first upcoming intersection 
for i = 2:length(Int_gap)
    Int_gap(i) = Int_dx(i)-Int_dx(i-1);         %   m - Distance between further intersections 
end
Int_out = [Int_cur,Int_dx,Int_gap];

== matlab function InfrastructureVariants_CL/Infrastructure v5/Signal Info v5/Cycle v5 ==
  data: Sig_out output; Int_out output; t_0 input; Sig_in input; Int_in input; hyp_out output; hyp input; Buffer input
function [Sig_out,Int_out,hyp_out] = fcn(t_0,Sig_in,Int_in,hyp,Buffer)

Int_cur = Int_in(~isnan(Int_in(:,1)),1);        %   Current intersections within communication range
Cs = Sig_in(:,:,1);                             %   s - Signal cycle start times
G = Sig_in(:,:,3);                              %   s - Signal green phase length 
R = Sig_in(:,:,4);                              %   s - Signal red phase length 
Y = Buffer(:,1);                                %   s - Signal yellow length
Rc = Buffer(:,2);                               %   s - Signal red clearance length 
N = 10;                                         %   # of upcoming intersections 
M = 20;                                         %   Size of intersection data queue
idx = zeros(N,1);                               %   Initialize current cycle index vector
Sig_out = NaN*ones(N,M,4);                      %   Initialize cycle length output 
hyp_out = NaN*ones(N,3,2);                      %   Initialize hyperparameter output 
T_0 = NaN*ones(N,1);                            %   Initialize current cycle start time output
L_0 = NaN*ones(N,1);                            %   Initialize light status flag
B_0 = NaN*ones(N,1);                            %   Initialize yellow light length 
for i = 1:length(Int_cur)
    idx(i) = find(Cs(Int_cur(i),:) <= t_0,1,'last');        %   Find current cycle for upcoming intersections 
    tR = Cs(Int_cur(i),idx(i))+G(Int_cur(i),idx(i));        %   s - Time at which light turns red
    tL1 = tR-t_0;                                           %   s - Time left until red
    tL2 = Cs(Int_cur(i),idx(i)+1)-t_0;                      %   s - Time left until green
    if tL1 > Y(Int_cur(i))*2 
        L_0(i) = 0;                                         %   Light is green and time left is unknown 
        Sig_out(i,:,3) = idx(i)-M:idx(i)-1;                 %   Available green phase lengths
        Sig_out(i,:,4) = idx(i)-M:idx(i)-1;                 %   Available red phase lengths
    elseif tL1 <= Y(Int_cur(i))*2 && tL1 > 0
        L_0(i) = 1;                                         %   Light is green and time left is known 
        Sig_out(i,:,3) = idx(i)-M+1:idx(i);                 %   Available green phase lengths
        Sig_out(i,:,4) = idx(i)-M:idx(i)-1;                 %   Available red phase lengths
    elseif tL2 > (Y(Int_cur(i))+Rc(Int_cur(i)))*2 
        L_0(i) = 2;                                         %   Light is red and time left is unknown 
        Sig_out(i,:,3) = idx(i)-M+1:idx(i);                 %   Available green phase lengths
        Sig_out(i,:,4) = idx(i)-M:idx(i)-1;                 %   Available red phase lengths
    else           
        L_0(i) = 3;                                         %   Light is red and time left is known 
        Sig_out(i,:,3) = idx(i)-M+1:idx(i);                 %   Available green phase lengths
        Sig_out(i,:,4) = idx(i)-M+1:idx(i);                 %   Available red phase lengths
    end
    B_0(i) = 2*Y(Int_cur(i));                               %   Yellow light length for upcoming intersections 
    Sig_out(i,:,1) = G(Int_cur(i),Sig_out(i,:,3));          %   Create a vector with the past green phase lengths
    Sig_out(i,:,2) = R(Int_cur(i),Sig_out(i,:,4));          %   Create a vector with the past red phase lengths
    T_0(i) = Cs(Int_cur(i),idx(i));                         %   Current cycle start time
    hypG1 = var(Sig_out(i,:,1));
    hypR1 = var(Sig_out(i,:,2));
    hyp_out(i,:,1) = [hypG1 1 .0625];                       %   Get relevant hyperparameters 
    hyp_out(i,:,2) = [hypR1 1 .0625];                       %   Get relevant hyperparameters 
end
Int_out = [Int_in, T_0, L_0, B_0];                          %   Update intersection variables

== matlab function InfrastructureVariants_CL/Infrastructure v5/Signal Info v5/IntFcn ==
  data: x_0 input; I_mode output; Int_ran input; Int_pos input; Int_out output
function [I_mode,Int_out]  = fcn(x_0,Int_ran,Int_pos)

Int_pos = Int_pos(:,1);                         %   Intersection Positions
[Int_0,~] = find(x_0-Int_pos < 0,1,'first');    %   First intersection within range
[Int_f,~] = find(x_0+Int_ran-Int_pos...         %   Last intersection within range
    > 0,1,'last');
Int_cur = NaN*ones(10,1);                       %   Initialize upcoming intersection vector 
Int_dx = NaN*ones(10,1);                        %   m - Initialize distance to upcoming intersections vector 
Int_gap = NaN*ones(10,1);                       %   m - Initialize distance between intersections vector 
if isempty(Int_0)
    I_mode = 0;                                 %   No upcoming intersection
elseif Int_pos(Int_0(1))-x_0 > Int_ran
    I_mode = 0;                                 %   No upcoming intersection
else
    I_0 = Int_0(1);     I_f = Int_f(1);
    Int_cur(1:I_f-I_0+1,1) = (I_0:I_f)';            %   Upcoming intersections
    I_mode = 1;                                 %   Approaching intersection
    Int_dx(1:I_f-I_0+1,1) = ...                 %   m - Distance to upcoming intersection 
        Int_pos(Int_cur(1:I_f-I_0+1,1))-x_0;
end
Int_gap(1) = Int_dx(1);                         %   m - Distance to first upcoming intersection 
for i = 2:length(Int_gap)
    Int_gap(i) = Int_dx(i)-Int_dx(i-1);         %   m - Distance between further intersections 
end
Int_out = [Int_cur,Int_dx,Int_gap];
